simulink model "fault_detection"  (R2017b)
settings: Solver=ode23tb  StartTime=0.0  StopTime=1  RelTol=1e-3  EnableMultiTasking=on
libraries: powerlib x19, powerlib_extras x4, dsparch4 x3
settings Model: Creator=CHEEKU  LastModifiedBy=cheeku.triven
settings DataIOCC: LimitDataPoints=on  SaveFormat=Array
settings OptimizationCC: ExpressionDepthLimit=2147483647  LifeSpan=inf
settings DebuggingCC: UnderspecifiedInitializationDetection=Classic  MergeDetectMultiDrivingBlocksExec=none  SolverPrmCheckMsg=warning  FcnCallInpInsideContextMsg=warning  StateNameClashWarn=warning  SFUnexpectedBacktrackingDiag=warning  SFNoUnconditionalDefaultTransitionDiag=warning  SFExecutionAtInitializationDiag=none
settings HardwareCC: ProdBitPerPointer=32  ProdBitPerSizeT=32  ProdBitPerPtrDiffT=32  ProdLargestAtomicFloat=None  ProdIntDivRoundTo=Undefined  ProdEndianess=Unspecified  ProdWordSize=32  ProdHWDeviceType=32-bit Generic
settings ModelReferenceCC: PropagateSignalLabelsOutOfModel=off
settings CodeAppCC: StateflowObjectComments=on
settings GRTTargetCC: TargetLangStandard=C89/C90 (ANSI)  GeneratePreprocessorConditionals=Disable all  CombineOutputUpdateFcns=off  GRTInterface=on
settings ConfigComp: CovMetricSettings=dw  CovHtmlReporting=on  CovSaveCumulativeToWorkspaceVar=on  CovSaveSingleToWorkspaceVar=on  CovExternalEMLEnable=off

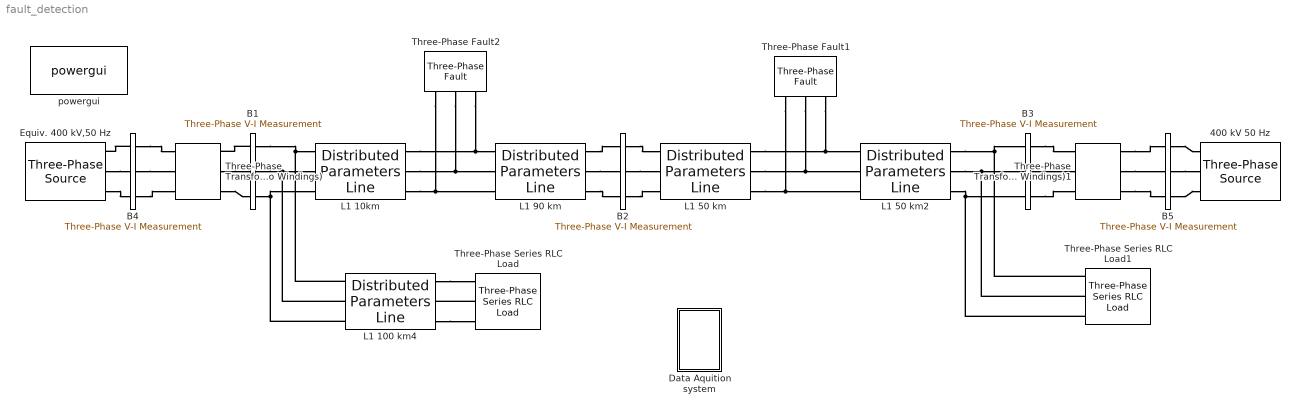
== system fault_detection ==
  400 kV 50 Hz : powerlib/Electrical Sources/Three-Phase Source  InternalConnection=Yg  VoltagePhases=off  Voltage=400e3  PhaseAngle=0  Voltage_phases=[25e3 25e3 25e3]/sqrt(3)  PhaseAngles_phases=[0 -120 +120]  Frequency=50  NonIdealSource=on  SpecifyImpedance=on  Resistance=0.8929  Inductance=16.58e-3  ShortCircuitLevel=1.2e12  BaseVoltage=400e3  XRratio=8  BusType=swing  Pref=10e3  Qref=0  Prefabc=[10e3, 10e3, 10e3]  Qrefabc=[0, 0, 0]  Qmin=-inf  Qmax=inf
  B1 : powerlib/Measurements/Three-Phase V-I Measurement  VoltageMeasurement=phase-to-ground  SetLabelV=on  LabelV=Vabc_B1  Vpu=off  VpuLL=off  CurrentMeasurement=yes  SetLabelI=on  LabelI=Iabc_B1  Ipu=off  Pbase=1.2e12  Vbase=400e3  OutputType=Complex  PhasorSimulation=off  PSBequivalent=0
  B2 : powerlib/Measurements/Three-Phase V-I Measurement  VoltageMeasurement=phase-to-ground  SetLabelV=on  LabelV=Vabc_B2  Vpu=off  VpuLL=off  CurrentMeasurement=yes  SetLabelI=on  LabelI=Iabc_B2  Ipu=off  Pbase=1.2e12  Vbase=400e3  OutputType=Complex  PhasorSimulation=off  PSBequivalent=0
  B3 : powerlib/Measurements/Three-Phase V-I Measurement  VoltageMeasurement=phase-to-ground  SetLabelV=on  LabelV=Vabc_B3  Vpu=on  VpuLL=off  CurrentMeasurement=yes  SetLabelI=on  LabelI=Iabc_B3  Ipu=on  Pbase=1.2e12  Vbase=400e3  OutputType=Complex  PhasorSimulation=off  PSBequivalent=0
  B4 : powerlib/Measurements/Three-Phase V-I Measurement  VoltageMeasurement=phase-to-ground  SetLabelV=on  LabelV=Vabc_B4  Vpu=off  VpuLL=off  CurrentMeasurement=yes  SetLabelI=on  LabelI=Iabc_B4  Ipu=off  Pbase=1.2e12  Vbase=400e3  OutputType=Complex  PhasorSimulation=off  PSBequivalent=0
  B5 : powerlib/Measurements/Three-Phase V-I Measurement  VoltageMeasurement=phase-to-ground  SetLabelV=on  LabelV=Vabc_B5  Vpu=off  VpuLL=off  CurrentMeasurement=yes  SetLabelI=on  LabelI=Iabc_B5  Ipu=off  Pbase=1.2e12  Vbase=400e3  OutputType=Complex  PhasorSimulation=off  PSBequivalent=0
  Data Aquition system : Subsystem
  Equiv. 400 kV,50 Hz : powerlib/Electrical Sources/Three-Phase Source  InternalConnection=Yg  VoltagePhases=off  Voltage=400e3  PhaseAngle=0  Voltage_phases=[25e3 25e3 25e3]/sqrt(3)  PhaseAngles_phases=[0 -120 +120]  Frequency=50  NonIdealSource=on  SpecifyImpedance=on  Resistance=0.8929  Inductance=16.58e-3  ShortCircuitLevel=1.2e12  BaseVoltage=400e3  XRratio=8  BusType=swing  Pref=10e3  Qref=0  Prefabc=[10e3, 10e3, 10e3]  Qrefabc=[0, 0, 0]  Qmin=-inf  Qmax=inf
  L1 100 km4 : powerlib/Elements/Distributed Parameters Line  Phases=3  Frequency=50  Resistance="[0.01755  0.2758]"  Inductance="[0.8737e-3  3.220e-3]"  Capacitance="[13.33e-9  8.297e-9]"  Length=100  x1=[-0.00052 3.81360932998659e-10 139869.056913819 -373511.570853464;-0.0005 3.84806328696385e-10 142213.122990857 -372625.380633916;-0.00048 3.88236532899147e-10 144551.574737307 -371724.479802378;-0.00046 3.91651410188359e-10 146884.319835099 -370808.903924871;-0.00044 3.9505082575051e-10 149211.266191449 -369878.689146763;-0.00042 3.98434645382497e-10 151532.321942501 -368933.872191342;-0.0004 4.01802735496913e-10 153847.395456948 -367974.490358363;-0.00038 4.05154963127328e-10 156156.395339651 -367000.581522578;-0.00036 4.08491195933535e-10 158459.230435248 -366012.184132239;-0.00034 4.11811302206776e-10 160755.809831754 -365009.337207585;-0.00032 4.15115150874939e-10 163046.042864145 -363992.080339294;-0.0003 4.18402611507737e-10 165329.839117944 -362960.453686925;-0.00028 4.21673554321853e-10 167607.108432785 -361914.497977332;-0.00026 4.24927850186065e-10 169877.760905973 -360854.254503056;-0.00024 4.28165370626344e-10 172141.706896039 -359779.765120694;-0.00022 4.31385987830928e-10 174398.85702627 -358691.072249246;-0.0002 4.34589574655363e-10 176649.122188244 -357588.218868444;-0.00018 4.37776004627527e-10 178892.413545346 -356471.24851705;-0.00016 4.40945151952622e-10 181128.642536275 -355340.205291141;-0.00014 4.44096891518136e-10 183357.720878537 -354195.133842366;-0.00012 4.47231098898789e-10 185579.560571939 -353036.079376187;-0.0001 4.50347650361439e-10 187794.073902052 -351863.087650089;-8e-05 4.53446422869972e-10 190001.173443682 -350676.204971776;-6e-05 4.56527294090155e-10 192200.772064319 -349475.478197345;-4e-05 4.59590142394467e-10 194392.782927575 -348260.954729433;-2e-05 4.62634846866901e-10 196577.119496615 -347032.682515346]  x2=[-0.00052 5.08780372544403e-10 136280.639600071 -373397.20297617;-0.0005 5.13374537366105e-10 138624.057919556 -372533.561556736;-0.00048 5.17948435040109e-10 140962.003598598 -371655.213150173;-0.00046 5.22501884996768e-10 143294.384339102 -370762.192432169;-0.00044 5.27034707473674e-10 145621.108062673 -369854.534657655;-0.00042 5.31546723522757e-10 147942.08291424 -368932.275659405;-0.0004 5.36037755017349e-10 150257.217265692 -367995.451846625;-0.00038 5.40507624659217e-10 152566.419719487 -367044.100203516;-0.00036 5.4495615598556e-10 154869.599112267 -366078.258287811;-0.00034 5.49383173375979e-10 157166.664518454 -365097.964229294;-0.00032 5.53788502059408e-10 159457.525253837 -364103.256728298;-0.0003 5.58171968121014e-10 161742.090879159 -363094.175054171;-0.00028 5.62533398509062e-10 164020.27120368 -362070.75904373;-0.00026 5.66872621041748e-10 166291.976288741 -361033.049099686;-0.00024 5.71189464413996e-10 168557.116451316 -359981.086189051;-0.00022 5.75483758204223e-10 170815.602267549 -358914.911841519;-0.0002 5.79755332881062e-10 173067.344576288 -357834.568147829;-0.00018 5.84004019810058e-10 175312.254482602 -356740.0977581;-0.00016 5.88229651260328e-10 177550.243361292 -355631.543880148;-0.00014 5.92432060411177e-10 179781.222860388 -354508.950277782;-0.00012 5.96611081358686e-10 182005.104904641 -353372.361269075;-0.0001 6.00766549122265e-10 184221.801698994 -352221.821724617;-8e-05 6.04898299651162e-10 186431.225732055 -351057.377065737;-6e-05 6.09006169830941e-10 188633.289779545 -349879.073262716;-4e-05 6.1308999748992e-10 190827.906907747 -348686.956832973;-2e-05 6.17149621405577e-10 193014.990476934 -347481.074839221]  x3=[-0.00052 -7.51911110948376e-13 461.362434287392 -1350.39824743861;-0.0005 -7.44737579962475e-13 469.838073987424 -1347.47278513841;-0.00048 -7.37534648012111e-13 478.295165284786 -1344.49412691989;-0.00046 -7.30302599456706e-13 486.733374307996 -1341.46239037538;-0.00044 -7.23041719805152e-13 495.152367931009 -1338.37769519265;-0.00042 -7.15752295704546e-13 503.551813786373 -1335.24016315018;-0.0004 -7.0843461492887e-13 511.931380278347 -1332.04991811237;-0.00038 -7.01088966367631e-13 520.290736595995 -1328.80708602463;-0.00036 -6.93715640014456e-13 528.629552726242 -1325.51179490841;-0.00034 -6.86314926955645e-13 536.947499466907 -1322.16417485617;-0.00032 -6.78887119358678e-13 545.244248439694 -1318.76435802622;-0.0003 -6.71432510460679e-13 553.51947210316 -1315.31247863749;-0.00028 -6.63951394556843e-13 561.772843765645 -1311.80867296429;-0.00026 -6.56444066988817e-13 570.004037598167 -1308.25307933085;-0.00024 -6.48910824133039e-13 578.212728647288 -1304.64583810593;-0.00022 -6.41351963389037e-13 586.398592847941 -1300.98709169723;-0.0002 -6.33767783167691e-13 594.561307036223 -1297.2769845458;-0.00018 -6.26158582879451e-13 602.700548962156 -1293.51566312031;-0.00016 -6.18524662922513e-13 610.815997302404 -1289.7032759113;-0.00014 -6.10866324670966e-13 618.907331672963 -1285.83997342528;-0.00012 -6.03183870462893e-13 626.974232641807 -1281.92590817882;-0.0001 -5.9547760358843e-13 635.016381741498 -1277.96123469251;-8e-05 -5.87747828277798e-13 643.03346148176 -1273.94610948488;-6e-05 -5.79994849689291e-13 651.025155362012 -1269.88069106618;-4e-05 -5.72218973897229e-13 658.991147883864 -1265.7651399322;-2e-05 -5.64420507879873e-13 666.931124563572 -1261.59961855782]  x4=[-0.00052 1.45046249862952e-12 455.739853508477 -1609.74723588471;-0.0005 1.44899414426036e-12 465.845131225169 -1606.851981742;-0.00048 1.44746858608347e-12 475.932018173734 -1603.89329183442;-0.00046 1.44588588432526e-12 486.000116141148 -1600.87128296599;-0.00044 1.44424610146809e-12 496.049027656143 -1597.78607444043;-0.00042 1.44254930224778e-12 506.078356004897 -1594.63778805651;-0.0004 1.44079555365105e-12 516.087705246702 -1591.42654810317;-0.00038 1.43898492491291e-12 526.076680229587 -1588.15248135467;-0.00036 1.43711748751386e-12 536.044886605924 -1584.81571706556;-0.00034 1.43519331517715e-12 545.991930847994 -1581.41638696558;-0.00032 1.4332124838658e-12 555.917420263522 -1577.95462525445;-0.0003 1.43117507177964e-12 565.820963011181 -1574.43056859662;-0.00028 1.42908115935221e-12 575.70216811606 -1570.84435611579;-0.00026 1.42693082924759e-12 585.560645485103 -1567.1961293895;-0.00024 1.42472416635712e-12 595.396005922502 -1563.4860324435;-0.00022 1.42246125779609e-12 605.207861145069 -1559.71421174604;-0.0002 1.42014219290024e-12 614.99582379756 -1555.88081620217;-0.00018 1.41776706322229e-12 624.759507467968 -1551.98599714777;-0.00016 1.41533596252829e-12 634.498526702782 -1548.02990834363;-0.00014 1.41284898679394e-12 644.212497022197 -1544.01270596935;-0.00012 1.41030623420076e-12 653.901034935297 -1539.93454861722;-0.0001 1.4077078051323e-12 663.563757955197 -1535.7955972859;-8e-05 1.40505380217007e-12 673.200284614135 -1531.5960153741;-6e-05 1.40234433008956e-12 682.81023447854 -1527.33596867413;-4e-05 1.39957949585611e-12 692.393228164047 -1523.01562536533;-2e-05 1.39675940862062e-12 701.948887350473 -1518.63515600746]  x5=0.000516878515707511  V1=[6.508e-11 4e+05 4e+05;314.2 314.2 314.2;0.9448 0.4163 -1.154]  V2=[2.374e-10 3.987e+05 3.987e+05;314.2 314.2 314.2;-1.856 0.408 -1.163]  I1=[2.491e-12 1431 1431;314.2 314.2 314.2;2.815 0.3872 -1.184]  I2=[3.385e-12 1678 1678;314.2 314.2 314.2;-0.2965 0.3339 -1.237]  nHarmo=1  Measurements=None
      settings: AttributesFormatString=\n  SourceProductName=Simscape Power Systems
  L1 10km : powerlib/Elements/Distributed Parameters Line  Phases=3  Frequency=50  Resistance="[0.01755  0.2758]"  Inductance="[0.8737e-3  3.220e-3]"  Capacitance="[13.33e-9  8.297e-9]"  Length=10  x1=[-6e-05 4.56527294090155e-10 0 0;-4e-05 4.59590142394467e-10 194392.782927575 -348260.954729433;-2e-05 4.62634846866901e-10 196577.119496615 -347032.682515346]  x2=[-6e-05 2.5288610101079e-10 0 0;-4e-05 2.56386088142962e-10 192644.901488578 -345166.841013994;-2e-05 2.59875953591377e-10 194809.831797382 -343949.612065779]  x3=[-6e-05 2.54560478280491e-12 0 0;-4e-05 2.27858697391763e-12 1833.39217801745 -657.92767582527;-2e-05 2.01147921031818e-12 1837.48984273163 -646.395221896411]  x4=[-6e-05 -6.73194815401354e-12 0 0;-4e-05 -6.49236286955511e-12 -336.908860263482 -2057.32091365618;-2e-05 -6.25252127772729e-12 -323.975766487165 -2059.39715077501]  x5=5.16878515707511e-05  V1=[7.276e-11 4e+05 4e+05;314.2 314.2 314.2;-0.9435 0.5128 -1.058]  V2=[9.092e-10 4.005e+05 4.005e+05;314.2 314.2 314.2;1.229 0.5128 -1.058]  I1=[7.394e-11 1570 1570;314.2 314.2 314.2;-0.04687 0.406 -1.165]  I2=[8.154e-11 1571 1571;314.2 314.2 314.2;3.114 0.6087 -0.962]  nHarmo=1  Measurements=None
      settings: AttributesFormatString=\n  SourceProductName=Simscape Power Systems
  L1 50 km : powerlib/Elements/Distributed Parameters Line  Phases=3  Frequency=50  Resistance="[0.01755  0.2758]"  Inductance="[0.8737e-3  3.220e-3]"  Capacitance="[13.33e-9  8.297e-9]"  Length=50  x1=[-0.00026 -6.72581206439265e-10 153852.163685321 -326918.285904644;-0.00024 -6.70253487940893e-10 155903.201430641 -325945.15752372;-0.00022 -6.67899308982475e-10 157948.084384518 -324959.161386084;-0.0002 -6.65518762502965e-10 159986.731818474 -323960.336417175;-0.00018 -6.63111942482263e-10 162019.063250198 -322948.722048894;-0.00016 -6.606789439375e-10 164044.998446727 -321924.358218043;-0.00014 -6.58219862919295e-10 166064.457427606 -320887.285364753;-0.00012 -6.55734796507954e-10 168077.360468055 -319837.544430883;-0.0001 -6.53223842809645e-10 170083.628102107 -318775.176858409;-8e-05 -6.5068710095252e-10 172083.181125751 -317700.224587783;-6e-05 -6.48124671082804e-10 174075.940600057 -316612.73005628;-4e-05 -6.45536654360842e-10 176061.827854295 -315512.736196322;-2e-05 -6.42923152957101e-10 178040.764489035 -314400.286433784]  x2=[-0.00026 -3.29727117125451e-10 145256.983619555 -308472.894605728;-0.00024 -3.25670275831412e-10 147192.295977339 -307554.1350748;-0.00022 -3.21600577632521e-10 149121.797435311 -306623.233833235;-0.0002 -3.17518183193492e-10 151045.411820058 -305680.227631422;-0.00018 -3.1342325368027e-10 152963.063190577 -304725.15369763;-0.00016 -3.09315950753659e-10 154874.675841276 -303758.049736543;-0.00014 -3.05196436562946e-10 156780.174304961 -302778.95392777;-0.00012 -3.01064873739497e-10 158679.483355815 -301787.904924336;-0.0001 -2.96921425390339e-10 160572.528012369 -300784.941851159;-8e-05 -2.92766255091717e-10 162459.233540462 -299770.104303505;-6e-05 -2.88599526882641e-10 164339.525456189 -298743.432345421;-4e-05 -2.84421405258404e-10 166213.329528845 -297704.966508159;-2e-05 -2.80232055164096e-10 168080.571783854 -296654.747788572]  x3=[-0.00026 -5.06063874307476e-12 1862.32147136276 -581.356073732496;-0.00024 -5.03012058035612e-12 1865.93745463783 -569.643364346598;-0.00022 -4.99940383708991e-12 1869.47977389719 -557.90816641606;-0.0002 -4.96848972592056e-12 1872.94828929613 -546.150943226404;-0.00018 -4.93737946728425e-12 1876.34286390362 -534.37215893267;-0.00016 -4.90607428936072e-12 1879.66336370765 -522.572278541093;-0.00014 -4.8745754280248e-12 1882.90965762059 -510.751767890746;-0.00012 -4.84288412679758e-12 1886.0816174843 -498.91109363515;-0.0001 -4.81100163679738e-12 1889.17911807524 -487.05072322385;-8e-05 -4.77892921669032e-12 1892.20203710939 -475.171124883961;-6e-05 -4.74666813264062e-12 1895.15025524708 -463.272767601686;-4e-05 -4.71421965826064e-12 1898.02365609772 -451.356121103795;-2e-05 -4.68158507456059e-12 1900.82212622435 -439.421655839089]  x4=[-0.00026 -2.63560219739492e-13 -763.419816114826 -1925.38770581052;-0.00024 -2.87743022048146e-13 -751.307258716123 -1930.14637691642;-0.00022 -3.11914464754984e-13 -739.16504099329 -1934.82884914829;-0.0002 -3.36073593612836e-13 -726.993642300293 -1939.43493765015;-0.00018 -3.60219454860663e-13 -714.793543143109 -1943.96446058153;-0.00016 -3.84351095261206e-13 -702.565225160765 -1948.41723912459;-0.00014 -4.08467562138623e-13 -690.309171106316 -1952.79309749129;-0.00012 -4.32567903416096e-13 -678.02586482779 -1957.09186293021;-0.0001 -4.56651167653416e-13 -665.715791249088 -1961.31336573346;-8e-05 -4.80716404084549e-13 -653.379436350834 -1965.45743924333;-6e-05 -5.04762662655168e-13 -641.017287151199 -1969.52391985891;-4e-05 -5.28788994060157e-13 -628.629831686663 -1973.5126470425;-2e-05 -5.52794449781092e-13 -616.21755899276 -1977.42346332598]  x5=0.000258439257853756  V1=[4.555e-10 4.023e+05 4.023e+05;314.2 314.2 314.2;0.3825 0.4695 -1.101]  V2=[1.204e-10 4.017e+05 4.017e+05;314.2 314.2 314.2;-0.3398 0.4696 -1.101]  I1=[7.338e-12 1567 1567;314.2 314.2 314.2;2.552 0.47 -1.101]  I2=[6.737e-12 1568 1568;314.2 314.2 314.2;-0.853 0.4155 -1.155]  nHarmo=1  Measurements=None
      settings: AttributesFormatString=\n  SourceProductName=Simscape Power Systems
  L1 50 km2 : powerlib/Elements/Distributed Parameters Line  Phases=3  Frequency=50  Resistance="[0.01755  0.2758]"  Inductance="[0.8737e-3  3.220e-3]"  Capacitance="[13.33e-9  8.297e-9]"  Length=50  x1=[-0.00026 -3.1567695022019e-10 145256.983619555 -308472.894605728;-0.00024 -3.11613159413915e-10 147192.295977339 -307554.1350748;-0.00022 -3.07537066653672e-10 149121.797435311 -306623.233833235;-0.0002 -3.03448832856627e-10 151045.411820058 -305680.227631422;-0.00018 -2.99348619419247e-10 152963.063190577 -304725.15369763;-0.00016 -2.9523658821094e-10 154874.675841276 -303758.049736543;-0.00014 -2.91112901567656e-10 156780.174304961 -302778.95392777;-0.00012 -2.86977722285484e-10 158679.483355815 -301787.904924336;-0.0001 -2.8283121361422e-10 160572.528012369 -300784.941851159;-8e-05 -2.78673539250928e-10 162459.233540462 -299770.104303505;-6e-05 -2.74504863333471e-10 164339.525456189 -298743.432345421;-4e-05 -2.70325350434038e-10 166213.329528845 -297704.966508159;-2e-05 -2.6613516555264e-10 168080.571783854 -296654.747788572]  x2=[-0.00026 -1.1044591613763e-10 136305.496650771 -289112.876605181;-0.00024 -1.09399693384622e-10 138119.343922971 -288250.742705764;-0.00022 -1.0834915171904e-10 139927.73847997 -287377.229160588;-0.0002 -1.07294332614473e-10 141730.60892945 -286492.370454474;-0.00018 -1.06235277713371e-10 143527.88409717 -285596.201520128;-0.00016 -1.05172028825409e-10 145319.493029785 -284688.757736765;-0.00014 -1.04104627925832e-10 147105.364997642 -283770.074928712;-0.00012 -1.030331171538e-10 148885.429497574 -282840.189363992;-0.0001 -1.01957538810724e-10 150659.616255682 -281899.137752897;-8e-05 -1.00877935358595e-10 152427.855230111 -280946.957246532;-6e-05 -9.97943494183089e-11 154190.076613814 -279983.685435353;-4e-05 -9.87068237679829e-11 155946.210837307 -279009.360347682;-2e-05 -9.76154013412678e-11 157696.18857142 -278024.020448204]  x3=[-0.00026 8.2859330146589e-12 1895.40385373495 -478.533840892711;-0.00024 8.31419283862268e-12 1898.37313710032 -466.61529975849;-0.00022 8.34212443248936e-12 1901.26747594478 -454.678337451209;-0.0002 8.36972669356746e-12 1904.08675600477 -442.723425221698;-0.00018 8.39699853216696e-12 1906.83086597996 -430.751035029424;-0.00016 8.42393887164237e-12 1909.49969753758 -418.761639523851;-0.00014 8.45054664843523e-12 1912.09314531673 -406.755712025784;-0.00012 8.47682081211606e-12 1914.61110693252 -394.733726508684;-0.0001 8.50276032542587e-12 1917.05348298016 -382.696157579954;-8e-05 8.52836416431709e-12 1919.42017703881 -370.643480462203;-6e-05 8.553631317994e-12 1921.71109567544 -358.576170974487;-4e-05 8.57856078895264e-12 1923.92614844851 -346.494705513521;-2e-05 8.60315159302018e-12 1926.06524791153 -334.399561034876]  x4=[-0.00026 -9.17831585940174e-12 -860.911613860711 -1879.0862785125;-0.00024 -9.18546030473002e-12 -849.088050590912 -1884.45841856963;-0.00022 -9.1922421238135e-12 -837.230966778746 -1889.7561634351;-0.0002 -9.19866104891757e-12 -825.340830521582 -1894.97930396302;-0.00018 -9.20471682663406e-12 -813.418111221638 -1900.12763395274;-0.00016 -9.21040921789124e-12 -801.463279567458 -1905.20095015702;-0.00014 -9.21573799796324e-12 -789.476807515325 -1910.19905229001;-0.00012 -9.22070295647895e-12 -777.459168270633 -1915.12174303519;-0.0001 -9.22530389743031e-12 -765.410836269201 -1919.96882805318;-8e-05 -9.22954063918005e-12 -753.332287158546 -1924.74011598935;-6e-05 -9.23341301446886e-12 -741.223997779106 -1929.43541848142;-4e-05 -9.236920870422e-12 -729.086446145412 -1934.0545501669;-2e-05 -9.24006406855531e-12 -716.92011142722 -1938.59732869036]  x5=0.000258439257853756  V1=[1.2e-10 4.017e+05 4.017e+05;314.2 314.2 314.2;-0.3262 0.4696 -1.101]  V2=[1.912e-10 4e+05 4e+05;314.2 314.2 314.2;0.835 0.4699 -1.101]  I1=[5.177e-12 1567 1567;314.2 314.2 314.2;0.2009 0.5237 -1.047]  I2=[3.73e-12 1567 1567;314.2 314.2 314.2;-2.117 0.3621 -1.209]  nHarmo=1  Measurements=None
      settings: AttributesFormatString=\n  SourceProductName=Simscape Power Systems
  L1 90 km : powerlib/Elements/Distributed Parameters Line  Phases=3  Frequency=50  Resistance="[0.01755  0.2758]"  Inductance="[0.8737e-3  3.220e-3]"  Capacitance="[13.33e-9  8.297e-9]"  Length=90  x1=[-0.00048 2.13409146303493e-10 143246.704423552 -368419.038428955;-0.00046 2.16753044009623e-10 145558.706714347 -367511.726486068;-0.00044 2.20088384676715e-10 147864.962596638 -366589.905809501;-0.00042 2.23415036631232e-10 150165.381023391 -365653.612791155;-0.0004 2.2673286854265e-10 152459.871178025 -364702.884394275;-0.00038 2.30041749428648e-10 154748.342477998 -363737.758151991;-0.00036 2.33341548660272e-10 157030.704578382 -362758.272165833;-0.00034 2.366321359671e-10 159306.867375429 -361764.465104232;-0.00032 2.3991338144238e-10 161576.741010129 -360756.376200989;-0.0003 2.43185155548157e-10 163840.235871757 -359734.045253728;-0.00028 2.46447329120393e-10 166097.262601413 -358697.512622322;-0.00026 2.49699773374061e-10 168347.732095545 -357646.819227308;-0.00024 2.5294235990823e-10 170591.555509472 -356582.006548259;-0.00022 2.56174960711137e-10 172828.644260887 -355503.116622158;-0.0002 2.59397448165237e-10 175058.910033356 -354410.192041732;-0.00018 2.62609695052243e-10 177282.264779806 -353303.275953771;-0.00016 2.65811574558148e-10 179498.620725998 -352182.412057428;-0.00014 2.69002960278232e-10 181707.890373995 -351047.64460249;-0.00012 2.72183726222051e-10 183909.986505614 -349899.018387633;-0.0001 2.75353746818412e-10 186104.822185869 -348736.578758653;-8e-05 2.78512896920329e-10 188292.310766408 -347560.371606676;-6e-05 2.81661051809967e-10 190472.365888925 -346370.443366346;-4e-05 2.8479808720356e-10 192644.901488578 -345166.841013994;-2e-05 2.87923879256323e-10 194809.831797382 -343949.612065779]  x2=[-0.00048 -7.09558939172392e-10 130907.857392127 -336762.804956973;-0.00046 -7.07447927258561e-10 133021.202568887 -335933.6446333;-0.00044 -7.05308986511906e-10 135129.296296339 -335091.222224549;-0.00042 -7.03142201374147e-10 137232.055350551 -334235.570988111;-0.0004 -7.00947657386249e-10 139329.396718197 -333366.724703635;-0.00038 -6.98725441185053e-10 141421.237599831 -332484.717671682;-0.00036 -6.96475640499848e-10 143507.495413156 -331589.58471238;-0.00034 -6.94198344148913e-10 145588.087796286 -330681.361164046;-0.00032 -6.9189364203601e-10 147662.932610997 -329760.082881791;-0.0003 -6.8956162514683e-10 149731.947945968 -328825.786236103;-0.00028 -6.87202385545409e-10 151795.052120016 -327878.508111415;-0.00026 -6.84816016370485e-10 153852.163685321 -326918.285904644;-0.00024 -6.82402611831827e-10 155903.201430641 -325945.15752372;-0.00022 -6.79962267206515e-10 157948.084384518 -324959.161386083;-0.0002 -6.77495078835175e-10 159986.731818474 -323960.336417175;-0.00018 -6.75001144118181e-10 162019.063250198 -322948.722048894;-0.00016 -6.72480561511803e-10 164044.998446727 -321924.358218043;-0.00014 -6.69933430524329e-10 166064.457427606 -320887.285364753;-0.00012 -6.67359851712127e-10 168077.360468055 -319837.544430883;-0.0001 -6.64759926675682e-10 170083.628102107 -318775.176858409;-8e-05 -6.62133758055584e-10 172083.181125751 -317700.224587783;-6e-05 -6.59481449528472e-10 174075.940600057 -316612.73005628;-4e-05 -6.56803105802946e-10 176061.827854295 -315512.736196322;-2e-05 -6.5409883261543e-10 178040.764489035 -314400.286433784]  x3=[-0.00048 -8.43022901331249e-13 1730.27315505941 -881.326506895626;-0.00046 -9.01408262403861e-13 1735.77650227217 -870.437554931936;-0.00044 -9.59758037421731e-13 1741.21132400074 -859.514239584005;-0.00042 -1.01806992283565e-12 1746.57740568768 -848.55699208562;-0.0004 -1.07634161659224e-12 1751.87453548926 -837.566245010149;-0.00038 -1.13457081822479e-12 1757.10250428386 -826.542432253468;-0.00036 -1.19275522894413e-12 1762.26110568024 -815.48598901683;-0.00034 -1.25089255172936e-12 1767.35013602564 -804.397351789681;-0.00032 -1.30898049141852e-12 1772.36939441386 -793.276958332432;-0.0003 -1.36701675479921e-12 1777.31868269317 -782.125247659175;-0.00028 -1.42499905069913e-12 1782.19780547414 -770.942660020354;-0.00026 -1.48292509007652e-12 1787.00657013736 -759.729636885381;-0.00024 -1.54079258611053e-12 1791.74478684105 -748.486620925209;-0.00022 -1.59859925429149e-12 1796.4122685285 -737.214055994857;-0.0002 -1.65634281251114e-12 1801.00883093554 -725.912387115887;-0.00018 -1.71402098115266e-12 1805.53429259776 -714.582060458835;-0.00016 -1.77163148318072e-12 1809.98847485768 -703.223523325597;-0.00014 -1.82917204423134e-12 1814.37120187181 -691.837224131769;-0.00012 -1.8866403927017e-12 1818.68230061759 -680.423612388948;-0.0001 -1.9440342598398e-12 1822.92160090022 -668.983138686981;-8e-05 -2.00135137983405e-12 1827.08893535939 -657.516254676181;-6e-05 -2.05858948990268e-12 1831.18413947587 -646.023413049495;-4e-05 -2.11574633038312e-12 1835.20705157801 -634.505067524631;-2e-05 -2.17281964482117e-12 1839.15751284814 -622.961672826148]  x4=[-0.00048 -1.04584390477988e-12 -796.95145260547 -1911.9467484341;-0.00046 -9.78859543587615e-13 -784.922684791202 -1916.91636895246;-0.00044 -9.11836538696643e-13 -772.86292957334 -1921.81031289485;-0.00042 -8.44777536060438e-13 -760.772663050373 -1926.62838705676;-0.0004 -7.776851830536e-13 -748.65236252532 -1931.37040122887;-0.00038 -7.10562128367344e-13 -736.502506486893 -1936.03616820457;-0.00036 -6.43411021904938e-13 -724.323574590603 -1940.62550378737;-0.00034 -5.76234514677084e-13 -712.11604763983 -1945.13822679817;-0.00032 -5.09035258697262e-13 -699.880407566834 -1949.57415908238;-0.0003 -4.41815906877034e-13 -687.617137413734 -1953.933125517;-0.00028 -3.74579112921313e-13 -675.326721313438 -1958.2149540175;-0.00026 -3.07327531223595e-13 -663.009644470529 -1962.41947554461;-0.00024 -2.40063816761174e-13 -650.666393142111 -1966.54652411102;-0.00022 -1.72790624990323e-13 -638.297454618611 -1970.59593678793;-0.0002 -1.05510611741462e-13 -625.903317204543 -1974.56755371146;-0.00018 -3.82264331143121e-14 -613.48447019923 -1978.46121808896;-0.00016 2.90592546269629e-14 -601.041403877487 -1982.27677620525;-0.00014 9.63437951586225e-14 -588.574609470267 -1986.01407742861;-0.00012 1.63624532202216e-13 -576.084579145266 -1989.6729742168;-0.0001 2.30898809629449e-13 -563.571805987495 -1993.25332212283;-8e-05 2.98163971567039e-13 -551.036783979813 -1996.7549798007;-6e-05 3.65417362501571e-13 -538.480007983426 -2000.17780901096;-4e-05 4.32656327384325e-13 -525.901973718349 -2003.52167462617;-2e-05 4.99878211736101e-13 -513.303177743838 -2006.78644463624]  x5=0.00046519066413676  V1=[9.158e-10 4.005e+05 4.005e+05;314.2 314.2 314.2;1.118 0.427 -1.144]  V2=[9.264e-10 4.023e+05 4.023e+05;314.2 314.2 314.2;0.1946 0.4267 -1.144]  I1=[8.175e-12 1564 1564;314.2 314.2 314.2;-2.54 0.3308 -1.24]  I2=[8.725e-12 1565 1565;314.2 314.2 314.2;0.7759 0.4262 -1.145]  nHarmo=1  Measurements=None
      settings: AttributesFormatString=\n  SourceProductName=Simscape Power Systems
  Three-Phase Series RLC Load : powerlib/Elements/Three-Phase Series RLC Load  LConnTagsString=A|B|C  Configuration=Y (grounded)  NominalVoltage=400e3  Vabc=[1e3 1e3 1e3]  Vabcp=[1e3 1e3 1e3]  NominalFrequency=50  UnbalancedPower=off  ActivePower=50e6  InductivePower=50e6  CapacitivePower=0  Pabc=[10e3 9e3 11e3]  QLabc=[100 90 110]  QCabc=[100 90 110]  Pabcp=[10e3 9e3 11e3]  QLabcp=[100 90 110]  QCabcp=[100 90 110]  Measurements=None  LoadType=constant Z
  Three-Phase Series RLC Load1 : powerlib/Elements/Three-Phase Series RLC Load  LConnTagsString=A|B|C  Configuration=Y (grounded)  NominalVoltage=400e3  Vabc=[1e3 1e3 1e3]  Vabcp=[1e3 1e3 1e3]  NominalFrequency=50  UnbalancedPower=off  ActivePower=100e6  InductivePower=100e6  CapacitivePower=0  Pabc=[10e3 9e3 11e3]  QLabc=[100 90 110]  QCabc=[100 90 110]  Pabcp=[10e3 9e3 11e3]  QLabcp=[100 90 110]  QCabcp=[100 90 110]  Measurements=None  LoadType=constant Z
  Three-Phase Transformer (Two Windings) : powerlib/Elements/Three-Phase Transformer (Two Windings)  Winding1Connection=Yg  Winding2Connection=Yg  CoreType=Three single-phase transformers  SetSaturation=off  Hysteresis=off  DataFile='hysteresis'  SetInitialFlux=off  Measurements=None  UNITS=pu  NominalPower=[ 1.2e12 , 50 ]  Winding1=[ 400e3 , 0.002 , 0.08 ]  Winding2=[ 400e3 , 0.002 , 0.08 ]  Rm=500  Lm=500  L0=0.5  Saturation=[ 0,0 ; 0.0024,1.2 ; 1.0,1.52 ]  InitialFluxes=[ 0.8 , -0.8 , 0.7 ]  MoreParameters=off  BreakLoop=off  DataType=off  TransfoNumber=1
  Three-Phase Transformer (Two Windings)1 : powerlib/Elements/Three-Phase Transformer (Two Windings)  Winding1Connection=Yg  Winding2Connection=Yg  CoreType=Three single-phase transformers  SetSaturation=off  Hysteresis=off  DataFile='hysteresis'  SetInitialFlux=off  Measurements=None  UNITS=pu  NominalPower=[ 1.2e12 , 50 ]  Winding1=[ 400e3 , 0.002 , 0.08 ]  Winding2=[ 500e3 , 0.002 , 0.08 ]  Rm=500  Lm=500  L0=0.5  Saturation=[ 0,0 ; 0.0024,1.2 ; 1.0,1.52 ]  InitialFluxes=[ 0.8 , -0.8 , 0.7 ]  MoreParameters=off  BreakLoop=off  DataType=off  TransfoNumber=1
  Three-Phase Fault1 : powerlib/Elements/Three-Phase Fault  InitialStates=0  FaultA=on  FaultB=off  FaultC=off  GroundFault=on  SwitchTimes=[2/10]  External=off  SwitchStatus=NaN  FaultResistance=0.001  GroundResistance=0.01  SnubberResistance=1e6  SnubberCapacitance=inf  Measurements=None
  Three-Phase Fault2 : powerlib/Elements/Three-Phase Fault  InitialStates=0  FaultA=on  FaultB=off  FaultC=off  GroundFault=on  SwitchTimes="[0.2   0.3]"  External=off  SwitchStatus=NaN  FaultResistance=0.001  GroundResistance=0.01  SnubberResistance=1e6  SnubberCapacitance=inf  Measurements=None
  powergui : powerlib/powergui  Priority=1  SimulationMode=Discrete  SampleTime=20e-6  frequency=60  Iterations=50  frequencyindice=50  Pbase=100e6  ErrMax=1e-4  UnitsV=kV  UnitsW=MW  buscounter=0  FunctionMessages=off  echomessages=off  EnableUseOfTLC=off  CurrentSourceSwitches=off  DisableSnubberDevices=off  DisableRonSwitches=off  DisableVfSwitches=off  DisplayEquations=off  SolverType=Tustin/Backward Euler (TBE)  Interpol=off  ExternalGateDelay=off  methode=off  Ts=100  x0status=blocks  SPID=off  SwTol=0  HookPort=off  RestoreLinks=warning  ResistiveCurrentMeasurement=off  Frange=[0:2:500]  Ylog=off  Xlog=on  ShowGrid=off  save=off  variable=ZData  structure=0  ZoomFFT=off  StartTime=0.0  cycles=1  DisplayStyle=1  fundamental=60  FreqAxis=off  MaxFrequency=1000  frequencyindicesteady=1  RmsSteady=1  display=off
  connections:
  B1/RConn1 -- L1 100 km4/LConn1 -- L1 10km/LConn1
  B1/RConn2 -- L1 100 km4/LConn2 -- L1 10km/LConn2
  B1/RConn3 -- L1 10km/LConn3 -- L1 100 km4/LConn3
  L1 10km/RConn1 -- Three-Phase Fault2/LConn1 -- L1 90 km/LConn1
  L1 10km/RConn2 -- L1 90 km/LConn2 -- Three-Phase Fault2/LConn2
  L1 10km/RConn3 -- Three-Phase Fault2/LConn3 -- L1 90 km/LConn3
  L1 90 km/RConn1 -- B2/LConn1
  L1 90 km/RConn2 -- B2/LConn2
  L1 90 km/RConn3 -- B2/LConn3
  B2/RConn1 -- L1 50 km/LConn1
  B2/RConn2 -- L1 50 km/LConn2
  B2/RConn3 -- L1 50 km/LConn3
  L1 50 km/RConn1 -- L1 50 km2/LConn1 -- Three-Phase Fault1/LConn1
  L1 50 km/RConn2 -- L1 50 km2/LConn2 -- Three-Phase Fault1/LConn2
  L1 50 km/RConn3 -- L1 50 km2/LConn3 -- Three-Phase Fault1/LConn3
  L1 100 km4/RConn1 -- Three-Phase Series RLC Load/LConn1
  L1 100 km4/RConn3 -- Three-Phase Series RLC Load/LConn3
  L1 50 km2/RConn1 -- Three-Phase Series RLC Load1/LConn1 -- B3/LConn1
  L1 50 km2/RConn2 -- Three-Phase Series RLC Load1/LConn2 -- B3/LConn2
  L1 50 km2/RConn3 -- Three-Phase Series RLC Load1/LConn3 -- B3/LConn3
  Three-Phase Transformer (Two Windings)/RConn2 -- B1/LConn2
  B1/LConn1 -- Three-Phase Transformer (Two Windings)/RConn1
  Three-Phase Transformer (Two Windings)/RConn3 -- B1/LConn3
  B4/LConn1 -- Equiv. 400 kV,50 Hz/RConn1
  Equiv. 400 kV,50 Hz/RConn2 -- B4/LConn2
  Equiv. 400 kV,50 Hz/RConn3 -- B4/LConn3
  B4/RConn1 -- Three-Phase Transformer (Two Windings)/LConn1
  B4/RConn2 -- Three-Phase Transformer (Two Windings)/LConn2
  B4/RConn3 -- Three-Phase Transformer (Two Windings)/LConn3
  B5/RConn1 -- 400 kV 50 Hz/RConn1
  B5/RConn2 -- 400 kV 50 Hz/RConn2
  B5/RConn3 -- 400 kV 50 Hz/RConn3
  Three-Phase Transformer (Two Windings)1/RConn1 -- B5/LConn1
  Three-Phase Transformer (Two Windings)1/RConn2 -- B5/LConn2
  Three-Phase Transformer (Two Windings)1/RConn3 -- B5/LConn3
  B3/RConn1 -- Three-Phase Transformer (Two Windings)1/LConn1
  B3/RConn2 -- Three-Phase Transformer (Two Windings)1/LConn2
  B3/RConn3 -- Three-Phase Transformer (Two Windings)1/LConn3
  Three-Phase Series RLC Load/LConn2 -- L1 100 km4/RConn2

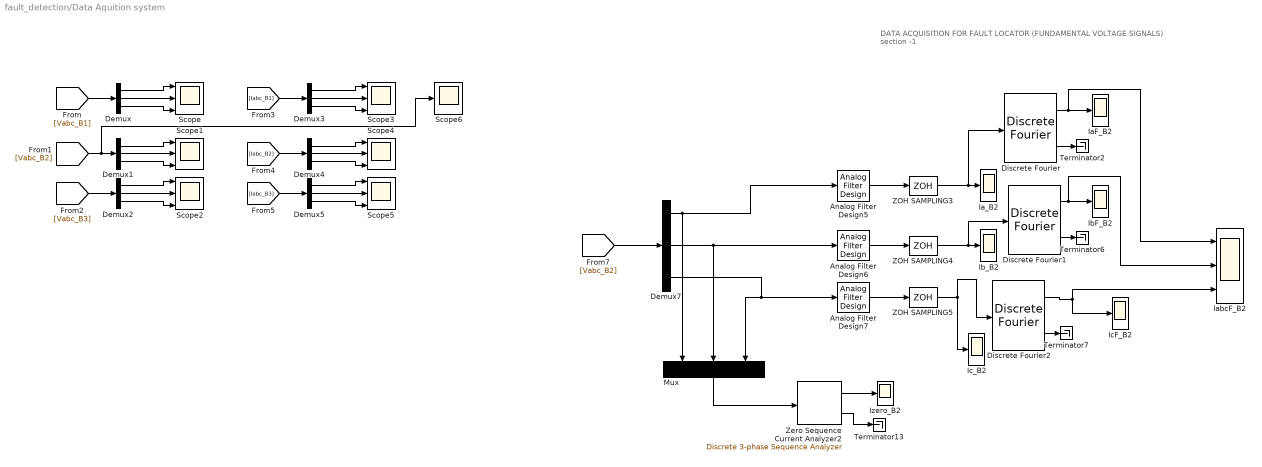
== system fault_detection/Data Aquition system ==
  note: DATA ACQUISITION FOR FAULT LOCATOR
      | (FUNDAMENTAL VOLTAGE SIGNALS) section -1
  " Izero_B2" : Scope
  Analog Filter Design5 : dsparch4/Analog Filter Design  method=Butterworth  filttype=Lowpass  N=2  Wlo=2*pi*400  Whi=80  Rp=2  Rs=40
  Analog Filter Design6 : dsparch4/Analog Filter Design  method=Butterworth  filttype=Lowpass  N=2  Wlo=2*pi*400  Whi=80  Rp=2  Rs=40
  Analog Filter Design7 : dsparch4/Analog Filter Design  method=Butterworth  filttype=Lowpass  N=2  Wlo=2*pi*400  Whi=80  Rp=2  Rs=40
  Demux{,1..5,7} (7 alike) : Demux  Outputs=3
  Discrete Fourier : powerlib_extras/Discrete Measurements/Discrete  Fourier  Freq=50  n=1  Par_Init=[0 0]  Ts=1e-3
  Discrete Fourier1 : powerlib_extras/Discrete Measurements/Discrete  Fourier  Freq=50  n=1  Par_Init=[0 0]  Ts=1e-3
  Discrete Fourier2 : powerlib_extras/Discrete Measurements/Discrete  Fourier  Freq=50  n=1  Par_Init=[0 0]  Ts=1e-3
  IaF_B2 : Scope
  Ia_B2 : Scope
  IabcF_B2 : Scope  NumInputPorts=3
  IbF_B2 : Scope
  Ib_B2 : Scope
  IcF_B2 : Scope
  Ic_B2 : Scope
  Mux : Mux  Inputs=3
  Scope{,1..5} (6 alike) : Scope  NumInputPorts=3
  Scope6 : Scope
  Terminator{2,6..7,13} (4 alike) : Terminator
  ZOH SAMPLING3 : ZeroOrderHold  SampleTime=1e-3
  ZOH SAMPLING4 : ZeroOrderHold  SampleTime=1e-3
  ZOH SAMPLING5 : ZeroOrderHold  SampleTime=1e-3
  Zero Sequence Current Analyzer2 : powerlib_extras/Discrete Measurements/Discrete 3-phase Sequence Analyzer  Freq=50  n=1  seq=Zero  Par_Init=[0 0]  Ts=1e-3
  wires:
  Demux/1 -> Scope/1
  Demux/3 -> Scope/3
  Demux/2 -> Scope/2
  [Vabc_B1] -> Demux/1
  Demux2/1 -> Scope2/1
  Demux2/2 -> Scope2/2
  Demux2/3 -> Scope2/3
  [Vabc_B3] -> Demux2/1
  Demux1/2 -> Scope1/2
  Demux1/1 -> Scope1/1
  [Vabc_B2] -> Scope6/1, Demux1/1
  Demux1/3 -> Scope1/3
  Demux5/3 -> Scope5/3
  Demux5/2 -> Scope5/2
  Demux5/1 -> Scope5/1
  [Iabc_B3] -> Demux5/1
  Demux3/2 -> Scope3/2
  Demux3/1 -> Scope3/1
  Demux4/2 -> Scope4/2
  Demux4/3 -> Scope4/3
  Demux3/3 -> Scope3/3
  [Iabc_B1] -> Demux3/1
  Demux4/1 -> Scope4/1
  Analog Filter Design6/1 -> ZOH SAMPLING4/1
  Discrete Fourier2/1 -> IcF_B2/1, IabcF_B2/3
  Mux/1 -> Zero Sequence Current Analyzer2/1
  ZOH SAMPLING3/1 -> Discrete Fourier/1, Ia_B2/1
  Demux7/2 -> Analog Filter Design6/1, Mux/2
  Discrete Fourier/1 -> IabcF_B2/1, IaF_B2/1
  [Vabc_B2] -> Demux7/1
  ZOH SAMPLING5/1 -> Ic_B2/1, Discrete Fourier2/1
  Discrete Fourier1/2 -> Terminator6/1
  Discrete Fourier/2 -> Terminator2/1
  Demux7/3 -> Analog Filter Design7/1, Mux/3
  Analog Filter Design7/1 -> ZOH SAMPLING5/1
  Demux7/1 -> Analog Filter Design5/1, Mux/1
  Zero Sequence Current Analyzer2/1 -> " Izero_B2"/1
  Analog Filter Design5/1 -> ZOH SAMPLING3/1
  ZOH SAMPLING4/1 -> Discrete Fourier1/1, Ib_B2/1
  Discrete Fourier2/2 -> Terminator7/1
  Discrete Fourier1/1 -> IabcF_B2/2, IbF_B2/1
  Zero Sequence Current Analyzer2/2 -> Terminator13/1
  [Iabc_B2] -> Demux4/1
